simulink model "Conventional_FSMPC_algorithm"  (R2019b)
settings: Solver=VariableStepAuto  StartTime=0.0  StopTime=0.1  FixedStep=1e-6  MaxStep=1  RelTol=1e-3
InitFcn:
  | %initialization file
  | clear
  | Rl=0.1;
  | Rload=60;
  | L=2.4e-3;
  | C=14e-6;
  | wref=2*pi*50;
  | Vdc=700;
  | Ts=20e-6;
  | s=tf('s');
  | Vac=325;
  | Td=4e-6;
  | 
  | 
  | % Converter states
  | v0 = 0;
  | v1 = 2/3*Vdc;
  | v2 = 1/3*Vdc + 1j*sqrt(3)/3*Vdc;
  | v3 = -1/3*Vdc + 1j*sqrt(3)/3*Vdc;
  | v4 = -2/3*Vdc;
  | v5 = -1/3*Vdc - 1j*sqrt(3)/3*Vdc;
  | v6 = 1/3*Vdc - 1j*sqrt(3)/3*Vdc;
  | v7 = 0;
  | v = [v0 v1 v2 v3 v4 v5 v6 v7];
  | states = [0 0 0;1 0 0;1 1 0;0 1 0;0 1 1;0 0 1;1 0 1;1 1 1];
  | 
  | %____________________________________________________________
  | % LC Filter model; x=[if,vc]; with linear load incoorporated;
  | Ac=[-Rl/L -1/L; 1/C -1/(Rload*C)];
  | Bc=[1/L,0;0,-1/C];
  | Cc=[0,1];
  | Dc=[0];
  | 
  | format long
  | % Discrete filter model - LC filter
  | system=ss(Ac,Bc,Cc,Dc);
  | systemd=c2d(system,Ts,'zoh');
  | Ad=systemd.a;
  | Bd=systemd.b;
  | Cd=systemd.c;
  | Dd=systemd.d;
  | 
  | %____________________________________________________________
  | 
  | % LC Filter model; x=[if,vc]; without load current as input;
  | Ac=[-Rl/L -1/L; 1/C 0];
  | Bc=[1/L,0;0,-1/C];
  | Cc=[0,1];
  | Dc=[0];
  | 
  | format long
  | % Discrete filter model - LC filter
  | system=ss(Ac,Bc,Cc,Dc);
  | systemd=c2d(system,Ts,'zoh');
  | Adf=systemd.a;
  | Bdf=systemd.b;
  | Cdf=systemd.c;
  | Ddf=systemd.d;
undefined symbols (not defined in the file): Lc, Lload, plecs
libraries: powerlib x19, powerlib_meascontrol x3
settings Model: Creator=Tomislav  LastModifiedBy=Kristina
settings DataIOCC: LimitDataPoints=on  ReturnWorkspaceOutputs=off
settings OptimizationCC: LifeSpan=inf
settings DebuggingCC: AllowSymbolicDim=off  SFUnexpectedBacktrackingDiag=warning  SFNoUnconditionalDefaultTransitionDiag=warning  SFExecutionAtInitializationDiag=none  ArithmeticOperatorsInVariantConditions=warning
settings ModelReferenceCC: PropagateSignalLabelsOutOfModel=off
settings SFSimCC: SimUseLocalCustomCode=off  CustomCodeUndefinedFunction=UseInterfaceOnly
settings RTWCC: RTWUseLocalCustomCode=off
settings CodeAppCC: StateflowObjectComments=on
settings GRTTargetCC: TargetLangStandard=C89/C90 (ANSI)
settings ConfigComp: CovMetricSettings=dw  CovHtmlReporting=on  CovSaveCumulativeToWorkspaceVar=on  CovSaveSingleToWorkspaceVar=on  CovExternalEMLEnable=off
settings SimscapeCC: SimscapeNormalizeSystem=off

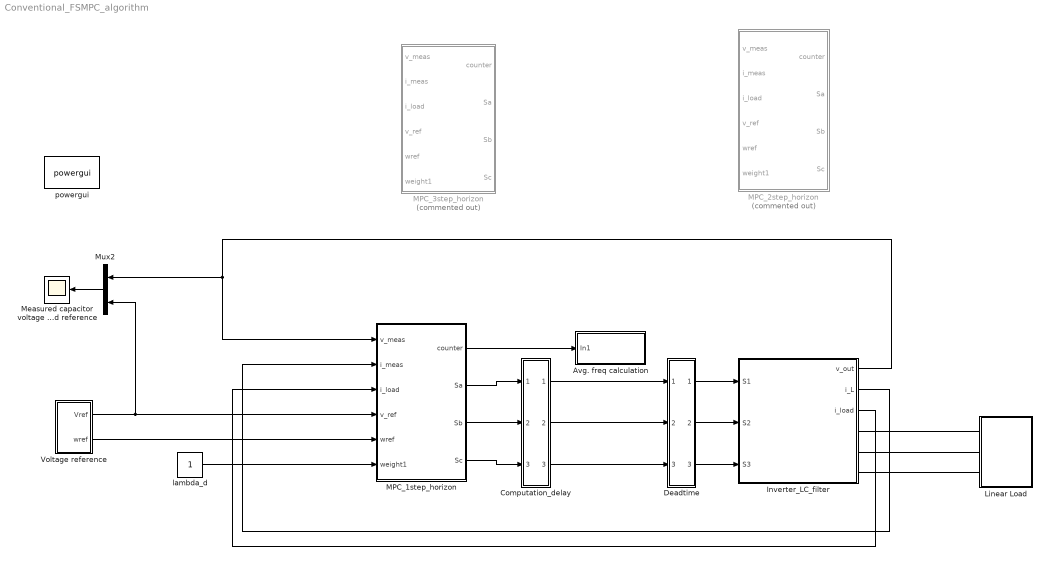
== system Conventional_FSMPC_algorithm ==
  Avg. freq calculation : Subsystem
  Computation_delay : Subsystem
  Deadtime : Subsystem
  Inverter_LC_filter : Subsystem
  Linear Load : Subsystem
  MPC_1step_horizon : MATLAB Function  TreatAsAtomicUnit=on
  MPC_2step_horizon : MATLAB Function  Commented=on  TreatAsAtomicUnit=on
  MPC_3step_horizon : MATLAB Function  Commented=on  TreatAsAtomicUnit=on  SystemSampleTime=Ts
  "Measured capacitor voltage and reference " : Scope
  Mux2 : Mux  Inputs=2
  Voltage reference : Subsystem
  lambda_d : Constant
  powergui : powerlib/powergui  Priority=1  SimulationMode=Continuous  SampleTime=1e-6  frequency=60  Iterations=50  frequencyindice=0  Pbase=100e6  ErrMax=1e-4  UnitsV=kV  UnitsW=MW  buscounter=0  FunctionMessages=off  echomessages=off  EnableUseOfTLC=off  CurrentSourceSwitches=off  DisableSnubberDevices=off  DisableRonSwitches=off  DisableVfSwitches=off  DisplayEquations=off  AutomaticDiscreteSolvers=off  SolverType=Tustin/Backward Euler (TBE)  Interpol=off  ExternalGateDelay=off  methode=off  Ts=100  x0status=blocks  SPID=off  SwTol=0  HookPort=off  NonlinearTolerance=1e-4  nMaxIteration=100  ContinueOnMaxIteration=off  RestoreLinks=warning  ResistiveCurrentMeasurement=off  Frange=[0:2:500]  Ylog=off  Xlog=on  ShowGrid=off  save=off  variable=ZData  structure=refs_2  ZoomFFT=off  StartTime=0.01  cycles=8  DisplayStyle=1  fundamental=50  FreqAxis=off  MaxFrequency=10000  frequencyindicesteady=1  RmsSteady=1  display=off
      settings: SourceProductName=Simscape Electrical
  wires:
  Mux2/1 -> "Measured capacitor voltage and reference "/1
  lambda_d/1 -> MPC_1step_horizon/6(weight1)
  MPC_1step_horizon/2(Sa) -> Computation_delay/1(1)
  MPC_1step_horizon/3(Sb) -> Computation_delay/2(2)
  MPC_1step_horizon/4(Sc) -> Computation_delay/3(3)
  MPC_1step_horizon/1(counter) -> Avg. freq calculation/1(In1)
  Inverter_LC_filter/1(v_out) -> MPC_1step_horizon/1(v_meas), Mux2/1
  Inverter_LC_filter/2(i_L) -> MPC_1step_horizon/2(i_meas)
  Inverter_LC_filter/3(i_load) -> MPC_1step_horizon/3(i_load)
  Voltage reference/1(Vref) -> MPC_1step_horizon/4(v_ref), Mux2/2
  Voltage reference/2(wref) -> MPC_1step_horizon/5(wref)
  Deadtime/3(S3) -> Inverter_LC_filter/3(S3)
  Deadtime/2(S2) -> Inverter_LC_filter/2(S2)
  Deadtime/1(S1) -> Inverter_LC_filter/1(S1)
  Computation_delay/1(S1) -> Deadtime/1(1)
  Computation_delay/2(S2) -> Deadtime/2(2)
  Computation_delay/3(S3) -> Deadtime/3(3)
  connections:
  Linear Load/LConn1 -- Inverter_LC_filter/RConn1
  Linear Load/LConn2 -- Inverter_LC_filter/RConn2
  Inverter_LC_filter/RConn3 -- Linear Load/LConn3

== system Conventional_FSMPC_algorithm/Avg. freq calculation ==
  In1 : Inport
  Discrete Transfer Fcn : DiscreteTransferFcn  Numerator=[0.0002]  Denominator=[1 -0.9998]
  Gain : Gain  Gain=1/(Ts*6)
  av_sw : Scope
  wires:
  Gain/1 -> av_sw/1
  In1/1 -> Discrete Transfer Fcn/1
  Discrete Transfer Fcn/1 -> Gain/1

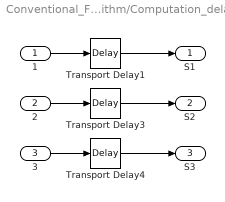
== system Conventional_FSMPC_algorithm/Computation_delay ==
  1 : Inport
  2 : Inport  Port=2
  3 : Inport  Port=3
  Transport Delay1 : TransportDelay  DelayTime=1*Ts
  Transport Delay3 : TransportDelay  DelayTime=1*Ts
  Transport Delay4 : TransportDelay  DelayTime=1*Ts
  S1 : Outport  VectorParamsAs1DForOutWhenUnconnected=off
  S2 : Outport  Port=2  VectorParamsAs1DForOutWhenUnconnected=off
  S3 : Outport  Port=3  VectorParamsAs1DForOutWhenUnconnected=off
  wires:
  2/1 -> Transport Delay3/1
  1/1 -> Transport Delay1/1
  3/1 -> Transport Delay4/1
  Transport Delay1/1 -> S1/1
  Transport Delay3/1 -> S2/1
  Transport Delay4/1 -> S3/1

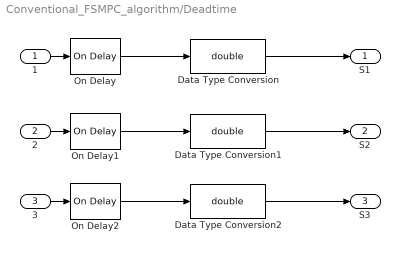
== system Conventional_FSMPC_algorithm/Deadtime ==
  1 : Inport
  2 : Inport  Port=2
  3 : Inport  Port=3
  Data Type Conversion : DataTypeConversion  OutDataTypeStr=double
  Data Type Conversion1 : DataTypeConversion  OutDataTypeStr=double
  Data Type Conversion2 : DataTypeConversion  OutDataTypeStr=double
  On Delay : powerlib_meascontrol/Logic/On Delay  DelayType=On delay  delay=4e-6  ic=0  Ts=0
      settings: SourceProductName=Simscape Electrical
  On Delay1 : powerlib_meascontrol/Logic/On Delay  DelayType=On delay  delay=4e-6  ic=0  Ts=0
      settings: SourceProductName=Simscape Electrical
  On Delay2 : powerlib_meascontrol/Logic/On Delay  DelayType=On delay  delay=4e-6  ic=0  Ts=0
      settings: SourceProductName=Simscape Electrical
  S1 : Outport  VectorParamsAs1DForOutWhenUnconnected=off
  S2 : Outport  Port=2  VectorParamsAs1DForOutWhenUnconnected=off
  S3 : Outport  Port=3  VectorParamsAs1DForOutWhenUnconnected=off
  wires:
  On Delay2/1 -> Data Type Conversion2/1
  3/1 -> On Delay2/1
  Data Type Conversion2/1 -> S3/1
  On Delay1/1 -> Data Type Conversion1/1
  2/1 -> On Delay1/1
  Data Type Conversion1/1 -> S2/1
  1/1 -> On Delay/1
  Data Type Conversion/1 -> S1/1
  On Delay/1 -> Data Type Conversion/1

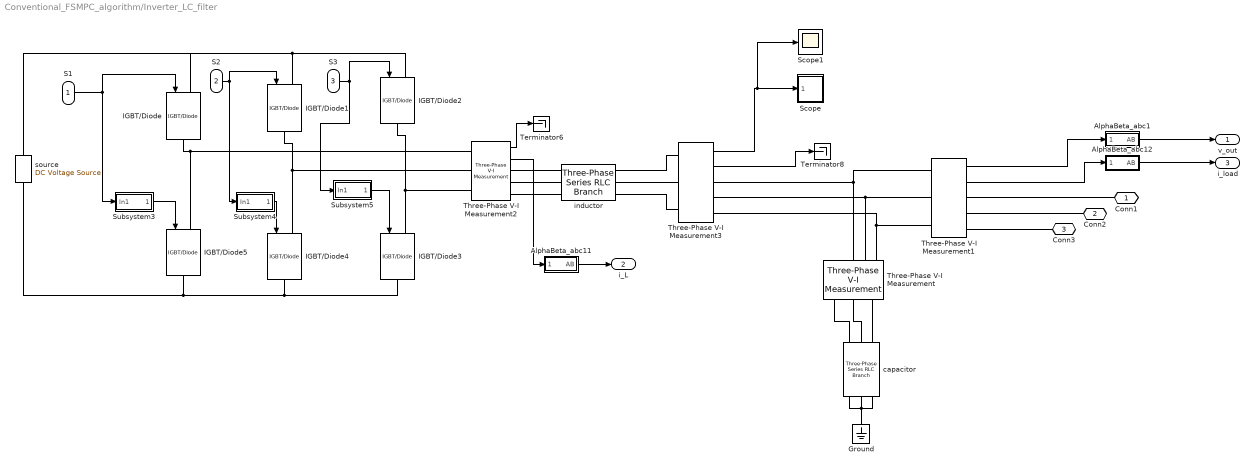
== system Conventional_FSMPC_algorithm/Inverter_LC_filter ==
  S1 : Inport
  S2 : Inport  Port=2
  S3 : Inport  Port=3
  AlphaBeta_abc1 : Subsystem
  AlphaBeta_abc11 : Subsystem
  AlphaBeta_abc12 : Subsystem
  Ground : powerlib/Elements/Ground  LConnTagsString=a
      settings: SourceProductName=Simscape Electrical
  IGBT/Diode{,1..5} (6 alike) : powerlib/Power Electronics/IGBT//Diode  Ron=1e-3  Rs=1e5  Cs=inf  Measurements=off
      settings: SourceProductName=Simscape Electrical
  Scope : Subsystem  LoadFcn=plecs('sl', 300);  InitFcn=plecs('sl', 314);  StartFcn=plecs('sl', 308);  StopFcn=plecs('sl', 309);  mask{Settings=<binary blob, 1008 chars, not shown>}
      mask init:
      | plecs('sl', 315);
      settings: CopyFcn=plecs('sl', 303);  DeleteFcn=plecs('sl', 305);  UndoDeleteFcn=plecs('sl', 306);  PreSaveFcn=plecs('sl', 311);  NameChangeFcn=plecs('sl', 310);  DestroyFcn=plecs('sl', 307);  OpenFcn=plecs('sl', 302);  ErrorFcn=plerrorfcn
      mask Display: plot([0.1 0.9 0.9 0.1 0.1], [0.9 0.9 0.5 0.5 0.9])
  Scope1 : Scope
  Subsystem3 : Subsystem
  Subsystem4 : Subsystem
  Subsystem5 : Subsystem
  Terminator6 : Terminator
  Terminator8 : Terminator
  Three-Phase V-I Measurement{,1..3} (4 alike) : powerlib/Measurements/Three-Phase V-I Measurement  VoltageMeasurement=phase-to-ground  SetLabelV=off  LabelV=Vabc  Vpu=off  VpuLL=off  CurrentMeasurement=yes  SetLabelI=off  LabelI=Iabc  Ipu=off  Pbase=100e6  Vbase=500e3  OutputType=Complex  PhasorSimulation=off  PSBequivalent=0
      settings: SourceProductName=Simscape Electrical
  capacitor : powerlib/Elements/Three-Phase Series RLC Branch  LConnTagsString=A|B|C  RConnTagsString=A|B|C  BranchType=C  Resistance=Rl  Inductance=Lc  Capacitance=C  Measurements=None
      settings: SourceProductName=Simscape Electrical
  inductor : powerlib/Elements/Three-Phase Series RLC Branch  LConnTagsString=A|B|C  RConnTagsString=A|B|C  BranchType=RL  Resistance=Rl  Inductance=L  Capacitance=1e-6  Measurements=None
      settings: SourceProductName=Simscape Electrical
  source : powerlib/Electrical Sources/DC Voltage Source  Amplitude=Vdc  Measurements=None
      settings: SourceProductName=Simscape Electrical
  Conn1 : PMIOPort  Side=Right
  Conn2 : PMIOPort  Port=2  Side=Right
  Conn3 : PMIOPort  Port=3  Side=Right
  v_out : Outport  VectorParamsAs1DForOutWhenUnconnected=off
  i_L : Outport  Port=2  VectorParamsAs1DForOutWhenUnconnected=off
  i_load : Outport  Port=3  VectorParamsAs1DForOutWhenUnconnected=off
  wires:
  Three-Phase V-I Measurement2/2 -> AlphaBeta_abc11/1(abc)
  Subsystem5/1(Out1) -> IGBT/Diode3/1
  S2/1 -> IGBT/Diode1/1, Subsystem4/1(In1)
  S1/1 -> IGBT/Diode/1, Subsystem3/1(In1)
  Subsystem4/1(Out1) -> IGBT/Diode4/1
  S3/1 -> IGBT/Diode2/1, Subsystem5/1(In1)
  Subsystem3/1(Out1) -> IGBT/Diode5/1
  AlphaBeta_abc11/1(AB) -> i_L/1
  Three-Phase V-I Measurement1/2 -> AlphaBeta_abc12/1(abc)
  AlphaBeta_abc12/1(AB) -> i_load/1
  Three-Phase V-I Measurement1/1 -> AlphaBeta_abc1/1(abc)
  AlphaBeta_abc1/1(AB) -> v_out/1
  Three-Phase V-I Measurement2/1 -> Terminator6/1
  Three-Phase V-I Measurement3/2 -> Terminator8/1
  Three-Phase V-I Measurement3/1 -> Scope1/1, Scope/1(1)
  connections:
  capacitor/RConn2 -- capacitor/RConn1 -- Ground/LConn1 -- capacitor/RConn3
  Three-Phase V-I Measurement/RConn3 -- Three-Phase V-I Measurement3/RConn3 -- Three-Phase V-I Measurement1/LConn3
  Three-Phase V-I Measurement2/RConn1 -- inductor/LConn1
  inductor/LConn2 -- Three-Phase V-I Measurement2/RConn2
  inductor/LConn3 -- Three-Phase V-I Measurement2/RConn3
  Three-Phase V-I Measurement/RConn1 -- Three-Phase V-I Measurement1/LConn1 -- Three-Phase V-I Measurement3/RConn1
  Three-Phase V-I Measurement/RConn2 -- Three-Phase V-I Measurement1/LConn2 -- Three-Phase V-I Measurement3/RConn2
  IGBT/Diode1/RConn1 -- IGBT/Diode4/LConn1 -- Three-Phase V-I Measurement2/LConn2
  IGBT/Diode2/RConn1 -- Three-Phase V-I Measurement2/LConn3 -- IGBT/Diode3/LConn1
  IGBT/Diode/RConn1 -- IGBT/Diode5/LConn1 -- Three-Phase V-I Measurement2/LConn1
  Three-Phase V-I Measurement1/RConn1 -- Conn1/RConn1
  Three-Phase V-I Measurement1/RConn2 -- Conn2/RConn1
  Three-Phase V-I Measurement1/RConn3 -- Conn3/RConn1
  capacitor/LConn1 -- Three-Phase V-I Measurement/LConn1
  capacitor/LConn2 -- Three-Phase V-I Measurement/LConn2
  capacitor/LConn3 -- Three-Phase V-I Measurement/LConn3
  inductor/RConn2 -- Three-Phase V-I Measurement3/LConn2
  inductor/RConn3 -- Three-Phase V-I Measurement3/LConn3
  inductor/RConn1 -- Three-Phase V-I Measurement3/LConn1
  IGBT/Diode1/LConn1 -- IGBT/Diode/LConn1 -- source/RConn1 -- IGBT/Diode2/LConn1
  IGBT/Diode5/RConn1 -- source/LConn1 -- IGBT/Diode3/RConn1 -- IGBT/Diode4/RConn1

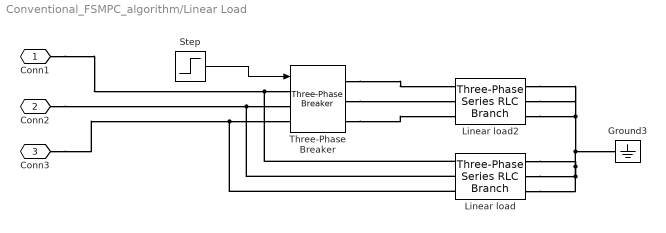
== system Conventional_FSMPC_algorithm/Linear Load ==
  Ground3 : powerlib/Elements/Ground  LConnTagsString=a
      settings: SourceProductName=Simscape Electrical
  Linear load : powerlib/Elements/Three-Phase Series RLC Branch  LConnTagsString=A|B|C  RConnTagsString=A|B|C  BranchType=R  Resistance=Rload  Inductance=1e-3  Capacitance=1e-6  Measurements=None
      settings: SourceProductName=Simscape Electrical
  Linear load2 : powerlib/Elements/Three-Phase Series RLC Branch  LConnTagsString=A|B|C  RConnTagsString=A|B|C  BranchType=R  Resistance=Rload  Inductance=Lload  Capacitance=1e-6  Measurements=None
      settings: SourceProductName=Simscape Electrical
  Step : Step  Time=0.025  Before=1  SampleTime=0
  Three-Phase Breaker : powerlib/Elements/Three-Phase Breaker  InitialState=open  SwitchA=on  SwitchB=on  SwitchC=on  SwitchTimes="[1/60  5/60]"  External=on  BreakerResistance=0.01  SnubberResistance=1e6  SnubberCapacitance=inf  Measurements=None
      settings: SourceProductName=Simscape Electrical
  Conn1 : PMIOPort  Side=Left
  Conn2 : PMIOPort  Port=2  Side=Left
  Conn3 : PMIOPort  Port=3  Side=Left
  wires:
  Step/1 -> Three-Phase Breaker/1
  connections:
  Three-Phase Breaker/RConn2 -- Linear load2/LConn2
  Linear load/RConn2 -- Linear load/RConn3 -- Linear load/RConn1 -- Linear load2/RConn3 -- Linear load2/RConn2 -- Linear load2/RConn1 -- Ground3/LConn1
  Three-Phase Breaker/RConn3 -- Linear load2/LConn3
  Three-Phase Breaker/RConn1 -- Linear load2/LConn1
  Conn1/RConn1 -- Linear load/LConn1 -- Three-Phase Breaker/LConn1
  Conn2/RConn1 -- Linear load/LConn2 -- Three-Phase Breaker/LConn2
  Conn3/RConn1 -- Linear load/LConn3 -- Three-Phase Breaker/LConn3

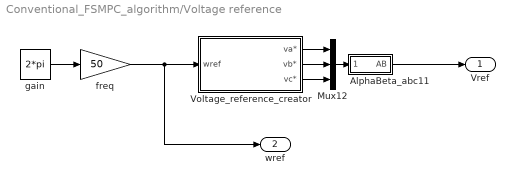
== system Conventional_FSMPC_algorithm/Voltage reference ==
  AlphaBeta_abc11 : Subsystem
  Mux12 : Mux  Inputs=3
  Voltage_reference_creator : Subsystem
  freq : Gain  Gain=50
  gain : Constant  Value=2*pi
  Vref : Outport  VectorParamsAs1DForOutWhenUnconnected=off
  wref : Outport  Port=2  VectorParamsAs1DForOutWhenUnconnected=off
  wires:
  Voltage_reference_creator/1(va*) -> Mux12/1
  AlphaBeta_abc11/1(AB) -> Vref/1
  Voltage_reference_creator/2(vb*) -> Mux12/2
  gain/1 -> freq/1
  Voltage_reference_creator/3(vc*) -> Mux12/3
  Mux12/1 -> AlphaBeta_abc11/1(abc)
  freq/1 -> wref/1, Voltage_reference_creator/1(wref)

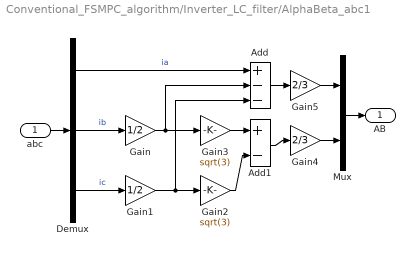
== system Conventional_FSMPC_algorithm/Inverter_LC_filter/AlphaBeta_abc1 ==
  abc : Inport
  Add : Sum  Inputs=+--
  Add1 : Sum  Inputs=+-
  Demux : Demux  Outputs=3
  Gain : Gain  Gain=1/2
  Gain1 : Gain  Gain=1/2
  Gain2 : Gain  Gain=sqrt(3)
  Gain3 : Gain  Gain=sqrt(3)
  Gain4 : Gain  Gain=2/3
  Gain5 : Gain  Gain=2/3
  Mux : Mux  Inputs=2
  AB : Outport  VectorParamsAs1DForOutWhenUnconnected=off
  wires:
  abc/1 -> Demux/1
  Gain/1 -> Gain3/1, Add/2
  Gain1/1 -> Gain2/1, Add/3
  Add1/1 -> Gain4/1
  Mux/1 -> AB/1
  Gain3/1 -> Add1/1
  Gain2/1 -> Add1/2
  Add/1 -> Gain5/1
  Demux/1 -> Add/1  "ia"
  Demux/2 -> Gain/1  "ib"
  Demux/3 -> Gain1/1  "ic"
  Gain5/1 -> Mux/1
  Gain4/1 -> Mux/2

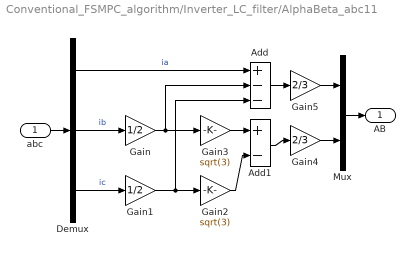
== system Conventional_FSMPC_algorithm/Inverter_LC_filter/AlphaBeta_abc11 ==
  abc : Inport
  Add : Sum  Inputs=+--
  Add1 : Sum  Inputs=+-
  Demux : Demux  Outputs=3
  Gain : Gain  Gain=1/2
  Gain1 : Gain  Gain=1/2
  Gain2 : Gain  Gain=sqrt(3)
  Gain3 : Gain  Gain=sqrt(3)
  Gain4 : Gain  Gain=2/3
  Gain5 : Gain  Gain=2/3
  Mux : Mux  Inputs=2
  AB : Outport  VectorParamsAs1DForOutWhenUnconnected=off
  wires:
  abc/1 -> Demux/1
  Gain/1 -> Gain3/1, Add/2
  Gain1/1 -> Gain2/1, Add/3
  Add1/1 -> Gain4/1
  Mux/1 -> AB/1
  Gain3/1 -> Add1/1
  Gain2/1 -> Add1/2
  Add/1 -> Gain5/1
  Demux/1 -> Add/1  "ia"
  Demux/2 -> Gain/1  "ib"
  Demux/3 -> Gain1/1  "ic"
  Gain5/1 -> Mux/1
  Gain4/1 -> Mux/2

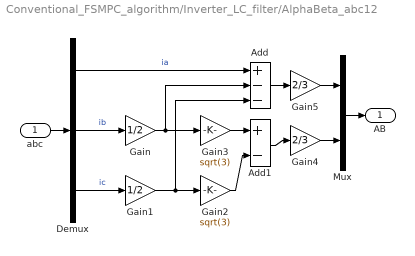
== system Conventional_FSMPC_algorithm/Inverter_LC_filter/AlphaBeta_abc12 ==
  abc : Inport
  Add : Sum  Inputs=+--
  Add1 : Sum  Inputs=+-
  Demux : Demux  Outputs=3
  Gain : Gain  Gain=1/2
  Gain1 : Gain  Gain=1/2
  Gain2 : Gain  Gain=sqrt(3)
  Gain3 : Gain  Gain=sqrt(3)
  Gain4 : Gain  Gain=2/3
  Gain5 : Gain  Gain=2/3
  Mux : Mux  Inputs=2
  AB : Outport  VectorParamsAs1DForOutWhenUnconnected=off
  wires:
  Gain4/1 -> Mux/2
  Gain5/1 -> Mux/1
  Demux/3 -> Gain1/1  "ic"
  Demux/2 -> Gain/1  "ib"
  Demux/1 -> Add/1  "ia"
  Add/1 -> Gain5/1
  Gain2/1 -> Add1/2
  Gain3/1 -> Add1/1
  Mux/1 -> AB/1
  Add1/1 -> Gain4/1
  Gain1/1 -> Add/3, Gain2/1
  Gain/1 -> Add/2, Gain3/1
  abc/1 -> Demux/1

== system Conventional_FSMPC_algorithm/Inverter_LC_filter/Scope ==
  1 : Inport
  " InputMux " : Subsystem
      mask Display: disp('Mux')
  " S-Function " : S-Function  FunctionName=plecs  SFunctionDeploymentMode=off  EnableBusSupport=off
  wires:
  1/1 -> " InputMux "/1(In1)
  " InputMux "/1(Out) -> " S-Function "/1

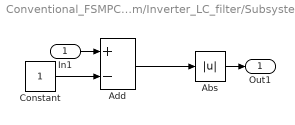
== system Conventional_FSMPC_algorithm/Inverter_LC_filter/Subsystem3 ==
  In1 : Inport
  Abs : Abs
  Add : Sum  Inputs=+-
  Constant : Constant
  Out1 : Outport  VectorParamsAs1DForOutWhenUnconnected=off
  wires:
  Constant/1 -> Add/2
  Abs/1 -> Out1/1
  In1/1 -> Add/1
  Add/1 -> Abs/1

== system Conventional_FSMPC_algorithm/Inverter_LC_filter/Subsystem4 ==
  In1 : Inport
  Abs : Abs
  Add : Sum  Inputs=+-
  Constant : Constant
  Out1 : Outport  VectorParamsAs1DForOutWhenUnconnected=off
  wires:
  Add/1 -> Abs/1
  In1/1 -> Add/1
  Abs/1 -> Out1/1
  Constant/1 -> Add/2

== system Conventional_FSMPC_algorithm/Inverter_LC_filter/Subsystem5 ==
  In1 : Inport
  Abs : Abs
  Add : Sum  Inputs=+-
  Constant : Constant
  Out1 : Outport  VectorParamsAs1DForOutWhenUnconnected=off
  wires:
  Constant/1 -> Add/2
  Abs/1 -> Out1/1
  In1/1 -> Add/1
  Add/1 -> Abs/1

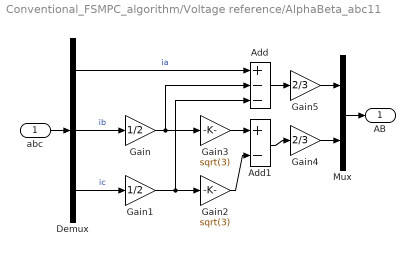
== system Conventional_FSMPC_algorithm/Voltage reference/AlphaBeta_abc11 ==
  abc : Inport
  Add : Sum  Inputs=+--
  Add1 : Sum  Inputs=+-
  Demux : Demux  Outputs=3
  Gain : Gain  Gain=1/2
  Gain1 : Gain  Gain=1/2
  Gain2 : Gain  Gain=sqrt(3)
  Gain3 : Gain  Gain=sqrt(3)
  Gain4 : Gain  Gain=2/3
  Gain5 : Gain  Gain=2/3
  Mux : Mux  Inputs=2
  AB : Outport  VectorParamsAs1DForOutWhenUnconnected=off
  wires:
  abc/1 -> Demux/1
  Gain/1 -> Gain3/1, Add/2
  Gain1/1 -> Gain2/1, Add/3
  Add1/1 -> Gain4/1
  Mux/1 -> AB/1
  Gain3/1 -> Add1/1
  Gain2/1 -> Add1/2
  Add/1 -> Gain5/1
  Demux/1 -> Add/1  "ia"
  Demux/2 -> Gain/1  "ib"
  Demux/3 -> Gain1/1  "ic"
  Gain5/1 -> Mux/1
  Gain4/1 -> Mux/2

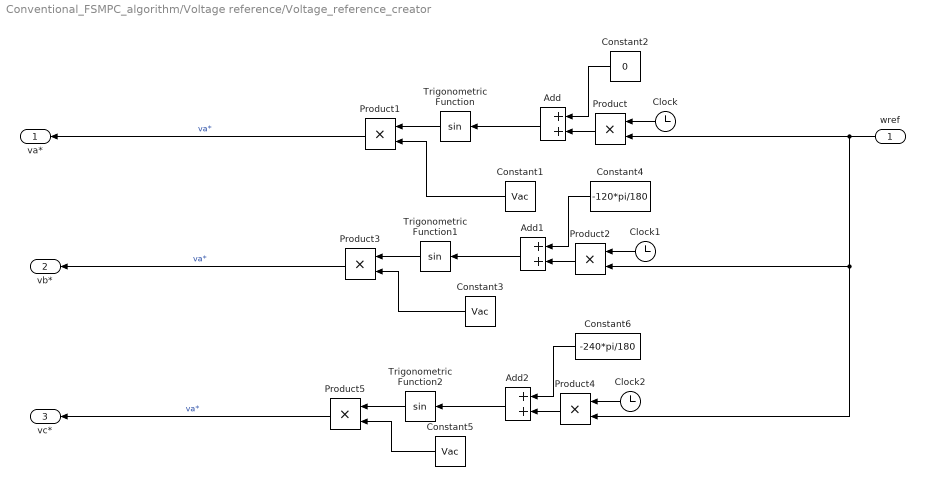
== system Conventional_FSMPC_algorithm/Voltage reference/Voltage_reference_creator ==
  wref : Inport
  Add : Sum
  Add1 : Sum
  Add2 : Sum
  Clock : Clock
  Clock1 : Clock
  Clock2 : Clock
  Constant1 : Constant  Value=Vac
  Constant2 : Constant  Value=0
  Constant3 : Constant  Value=Vac
  Constant4 : Constant  Value=-120*pi/180
  Constant5 : Constant  Value=Vac
  Constant6 : Constant  Value=-240*pi/180
  Product{,1..5} (6 alike) : Product
  Trigonometric Function : Trigonometry
  Trigonometric Function1 : Trigonometry
  Trigonometric Function2 : Trigonometry
  va* : Outport  VectorParamsAs1DForOutWhenUnconnected=off
  vb* : Outport  Port=2  VectorParamsAs1DForOutWhenUnconnected=off
  vc* : Outport  Port=3  VectorParamsAs1DForOutWhenUnconnected=off
  wires:
  Product1/1 -> va*/1  "va*"
  Add/1 -> Trigonometric Function/1
  Constant2/1 -> Add/1
  wref/1 -> Product/2, Product2/2, Product4/2
  Trigonometric Function/1 -> Product1/1
  Product/1 -> Add/2
  Clock/1 -> Product/1
  Product3/1 -> vb*/1  "va*"
  Add1/1 -> Trigonometric Function1/1
  Constant4/1 -> Add1/1
  Trigonometric Function1/1 -> Product3/1
  Product2/1 -> Add1/2
  Clock1/1 -> Product2/1
  Product5/1 -> vc*/1  "va*"
  Add2/1 -> Trigonometric Function2/1
  Constant6/1 -> Add2/1
  Trigonometric Function2/1 -> Product5/1
  Product4/1 -> Add2/2
  Clock2/1 -> Product4/1
  Constant1/1 -> Product1/2
  Constant3/1 -> Product3/2
  Constant5/1 -> Product5/2

== system Conventional_FSMPC_algorithm/Inverter_LC_filter/Scope/ InputMux  ==
  In1 : Inport
  Convert1 : DataTypeConversion  SaturateOnIntegerOverflow=on  RndMeth=Zero
  Mux : Mux  Inputs=1
  Out : Outport
  wires:
  Convert1/1 -> Mux/1
  In1/1 -> Convert1/1
  Mux/1 -> Out/1

== matlab function Conventional_FSMPC_algorithm/MPC_2step_horizon ==
  settings: updateMethod=DISCRETE  sampleTime=Ts
  data: counter output; Adf parameter; Bdf parameter; v parameter; states parameter; Sa output; Sb output; Sc output; v_meas input size=[1 2]; i_meas input size=[1 2]; i_load input; v_ref input; C parameter; wref input; weight1 input
function [counter,Sa,Sb,Sc] = fcn(Adf,Bdf,v,states,v_meas,i_meas,i_load, v_ref, C, wref, weight1)
%#codegen
persistent vc_old ift_old x_old v_ref_old v_ref_old2
% Initialize values
if isempty(vc_old), vc_old = 0+1j*0; end
if isempty(ift_old), ift_old = 0+1j*0; end
if isempty(x_old), x_old = 1; end
if isempty(v_ref_old), v_ref_old = 0+1j*0; end
if isempty(v_ref_old2), v_ref_old2 = 0+1j*0; end

g = zeros(8,8);

v_ref = v_ref(1) + 1j*v_ref(2);
v_ref1= 3*v_ref - 3*v_ref_old +v_ref_old2;

v_meas = v_meas(1) + 1j*v_meas(2);
i_meas = i_meas(1) + 1j*i_meas(2);
i_load = i_load(1) + 1j*i_load(2);

v_ref_old=v_ref;
v_ref_old2=v_ref_old;

% delay compensation
    iftd= Adf(1,1)*i_meas+Adf(1,2)*v_meas+Bdf(1,1)*v(x_old)+Bdf(1,2)*i_load;
    vcd=Adf(2,1)*i_meas+Adf(2,2)*v_meas+Bdf(2,1)*v(x_old)+Bdf(2,2)*i_load;  
    
for i = 1:8
    % N= 1 horizon       
        v_o1 = v(i);
        ift1= Adf(1,1)*iftd+Adf(1,2)*vcd+Bdf(1,1)*v_o1+Bdf(1,2)*i_load;
        vc1=Adf(2,1)*iftd+Adf(2,2)*vcd+Bdf(2,1)*v_o1+Bdf(2,2)*i_load;   
                 
        if sqrt(real(ift1)^2+imag(ift1)^2)>40
        constraint1=inf;
        else
        constraint1=0;
        end
        
        
   for j= 1:8
         % N= 2 horizon
         v_o2 = v(j);
         ift2= Adf(1,1)*ift1+Adf(1,2)*vc1+Bdf(1,1)*v_o2 +Bdf(1,2)*i_load;
         vc2=Adf(2,1)*ift1+Adf(2,2)*vc1+Bdf(2,1)*v_o2 + Bdf(2,2)*i_load;   
           
          
        if sqrt(real(ift2)^2+imag(ift2)^2)>40
        constraint2=inf;
        else
        constraint2=0;
        end  
        
        %Cost function     
        g(i,j) = (real(v_ref - vc1))^2+(imag(v_ref - vc1))^2 + (real(v_ref1 - vc2))^2+(imag(v_ref1 - vc2))^2 + constraint1 + constraint2 +weight1*((real(ift1 - i_load)+C*wref*imag(v_ref))^2+(imag(ift1 - i_load)-C*wref*real(v_ref))^2) + weight1*((real(ift2 - i_load)+C*wref*imag(v_ref1))^2+(imag(ift2 - i_load)-C*wref*real(v_ref1))^2);  
        
  end    
          
end


[M,I] = min(g(:));
[I_row, I_col] = ind2sub(size(g),I);

x_opt=I_row;

counter= sum(abs(states(x_opt,:)-states(x_old,:)));

x_old=x_opt;

Sa = states(x_opt,1);
Sb = states(x_opt,2);
Sc = states(x_opt,3);

== matlab function Conventional_FSMPC_algorithm/MPC_3step_horizon ==
  settings: updateMethod=DISCRETE  sampleTime=Ts
  data: counter output; Adf parameter; Bdf parameter; v parameter; states parameter; Sa output; Sb output; Sc output; v_meas input size=[1 2]; i_meas input size=[1 2]; i_load input; v_ref input; C parameter; wref input; weight1 input
function [counter,Sa,Sb,Sc] = fcn(Adf,Bdf,v,states,v_meas,i_meas,i_load, v_ref, C, wref, weight1)
%#codegen
persistent vc_old ift_old x_old v_ref_old v_ref_old2 
% Initialize values
if isempty(vc_old), vc_old = 0+1j*0; end
if isempty(ift_old), ift_old = 0+1j*0; end
if isempty(x_old), x_old = 1; end
if isempty(v_ref_old), v_ref_old = 0+1j*0; end
if isempty(v_ref_old2), v_ref_old2 = 0+1j*0; end

g = zeros(8,8,8);

v_ref = v_ref(1) + 1j*v_ref(2);
v_ref1= 3*v_ref - 3*v_ref_old +v_ref_old2;
v_ref2 = 6*v_ref - 8*v_ref_old + 3*v_ref_old2;

v_meas = v_meas(1) + 1j*v_meas(2);
i_meas = i_meas(1) + 1j*i_meas(2);
i_load = i_load(1) + 1j*i_load(2);

v_ref_old=v_ref;
v_ref_old2=v_ref_old;

% delay compensation
    iftd= Adf(1,1)*i_meas+Adf(1,2)*v_meas+Bdf(1,1)*v(x_old)+Bdf(1,2)*i_load;
    vcd=Adf(2,1)*i_meas+Adf(2,2)*v_meas+Bdf(2,1)*v(x_old)+Bdf(2,2)*i_load;  
    
for i = 1:8
     % N= 1 horizon   
    v_o1 = v(i);
    ift1= Adf(1,1)*iftd+Adf(1,2)*vcd+Bdf(1,1)*v_o1+Bdf(1,2)*i_load;
    vc1=Adf(2,1)*iftd+Adf(2,2)*vcd+Bdf(2,1)*v_o1+Bdf(2,2)*i_load;   
    
             
    if sqrt(real(ift1)^2+imag(ift1)^2)>40
        constraint1=inf;
    else
        constraint1=0;
    end
     
     % N= 2 horizon         
    for j= 1:8
         v_o2 = v(j);
           ift2= Adf(1,1)*ift1+Adf(1,2)*vc1+Bdf(1,1)*v_o2 +Bdf(1,2)*i_load;
           vc2=Adf(2,1)*ift1+Adf(2,2)*vc1+Bdf(2,1)*v_o2 + Bdf(2,2)*i_load;   
           
          
        if sqrt(real(ift2)^2+imag(ift2)^2)>40
        constraint2=inf;
    else
        constraint2=0;
        end  
     
       % N= 3 horizon     
    for k= 1:8
         v_o3 = v(k);
           ift3= Adf(1,1)*ift2+Adf(1,2)*vc2+Bdf(1,1)*v_o3 +Bdf(1,2)*i_load;
           vc3=Adf(2,1)*ift2+Adf(2,2)*vc2+Bdf(2,1)*v_o3 + Bdf(2,2)*i_load;   
           
          
        if sqrt(real(ift3)^2+imag(ift3)^2)>40
        constraint3=inf;
    else
        constraint3=0;
        end  
        
        
        %Cost function     
         g(i,j,k) = (real(v_ref - vc1))^2+(imag(v_ref - vc1))^2 + (real(v_ref1 - vc2))^2+(imag(v_ref1 - vc2))^2 +weight1*((real(ift1 - i_load)+C*wref*imag(v_ref))^2+(imag(ift1 - i_load)-C*wref*real(v_ref))^2) + weight1*((real(ift2 - i_load)+C*wref*imag(v_ref1))^2+(imag(ift2 - i_load)-C*wref*real(v_ref1))^2)+ (real(v_ref2 - vc3))^2+(imag(v_ref2 - vc3))^2 + weight1*((real(ift3 - i_load)+C*wref*imag(v_ref2))^2+(imag(ift3 - i_load)-C*wref*real(v_ref2))^2) + constraint1 + constraint2 +constraint3;  
        
         
    end   
     end    
          
end


[~,I] = min(g(:));
[I_row,~,~] = ind2sub(size(g),I);

x_opt=I_row;

counter= sum(abs(states(x_opt,:)-states(x_old,:)));

x_old=x_opt;

Sa = states(x_opt,1);
Sb = states(x_opt,2);
Sc = states(x_opt,3);

== matlab function Conventional_FSMPC_algorithm/MPC_1step_horizon ==
  settings: updateMethod=DISCRETE  sampleTime=Ts
  data: counter output; Adf parameter; Bdf parameter; v parameter; states parameter; Sa output; Sb output; Sc output; v_meas input size=[1 2]; i_meas input size=[1 2]; i_load input; v_ref input; C parameter; wref input; weight1 input
function [counter,Sa,Sb,Sc] = fcn(Adf,Bdf,v,states,v_meas,i_meas,i_load, v_ref, C, wref, weight1)
%#codegen
persistent vc_old ift_old x_old 
% Initialize values
if isempty(vc_old), vc_old = 0+1j*0; end
if isempty(ift_old), ift_old = 0+1j*0; end
if isempty(x_old), x_old = 1; end

g = zeros(1,8);

v_ref = v_ref(1) + 1j*v_ref(2);

v_meas = v_meas(1) + 1j*v_meas(2);
i_meas = i_meas(1) + 1j*i_meas(2);
i_load = i_load(1) + 1j*i_load(2);


% delay compensation
    iftd= Adf(1,1)*i_meas+Adf(1,2)*v_meas+Bdf(1,1)*v(x_old)+Bdf(1,2)*i_load;
    vcd=Adf(2,1)*i_meas+Adf(2,2)*v_meas+Bdf(2,1)*v(x_old)+Bdf(2,2)*i_load;  
    
for i = 1:8
     % N= 1 horizon     
    v_o1 = v(i);
    ift1= Adf(1,1)*iftd+Adf(1,2)*vcd+Bdf(1,1)*v_o1+Bdf(1,2)*i_load;
    vc1=Adf(2,1)*iftd+Adf(2,2)*vcd+Bdf(2,1)*v_o1+Bdf(2,2)*i_load;   
    
            
        if sqrt(real(ift1)^2+imag(ift1)^2)>40
        constraint1=inf;
        else
        constraint1=0;
        end
       
      %Cost function    
    g(i) = constraint1 + (real(v_ref - vc1))^2+(imag(v_ref - vc1))^2+  weight1*((real(ift1 - i_load)+C*wref*imag(v_ref))^2+(imag(ift1 - i_load)-C*wref*real(v_ref))^2);
end


[~,x_opt] = min(g);

counter= sum(abs(states(x_opt,:)-states(x_old,:)));

x_old=x_opt;

Sa = states(x_opt,1);
Sb = states(x_opt,2);
Sc = states(x_opt,3);
